simulink model "proc_control_lite"  (R2024b)
settings: Solver=FixedStepAuto  StartTime=0.0  StopTime=inf  RelTol=1e-3
InitFcn:
  | InitProcControl;
StartFcn:
  | LoadParams;
model workspace (MAT data in the model file):
  SL_ROS_VariableLengthArrays_MaxSizes.CommonInfo.ArrayTruncateAction = 'EmitWarning'
  SL_ROS_VariableLengthArrays_MaxSizes.MsgTypeMap = containers.Map
  SL_ROS_VariableLengthArrays_MaxSizes.MsgTypeMap.serialization.keys = {'sensor_msgs/Image', 'trajectory_msgs/MultiDOFJointTrajectoryPoint'}
  SL_ROS_VariableLengthArrays_MaxSizes.MsgTypeMap.serialization.values{1}(1).PropertyName = 'data'
  SL_ROS_VariableLengthArrays_MaxSizes.MsgTypeMap.serialization.values{1}(1).DataType = 'uint8'
  SL_ROS_VariableLengthArrays_MaxSizes.MsgTypeMap.serialization.values{1}(1).MaxLength = 2764800
  SL_ROS_VariableLengthArrays_MaxSizes.MsgTypeMap.serialization.values{1}(2).PropertyName = 'encoding'
  SL_ROS_VariableLengthArrays_MaxSizes.MsgTypeMap.serialization.values{1}(2).DataType = 'uint8'
  SL_ROS_VariableLengthArrays_MaxSizes.MsgTypeMap.serialization.values{1}(2).MaxLength = 128
  SL_ROS_VariableLengthArrays_MaxSizes.MsgTypeMap.serialization.values{2}(1).PropertyName = 'accelerations'
  SL_ROS_VariableLengthArrays_MaxSizes.MsgTypeMap.serialization.values{2}(1).DataType = 'geometry_msgs/Twist'
  SL_ROS_VariableLengthArrays_MaxSizes.MsgTypeMap.serialization.values{2}(1).MaxLength = 1024
  SL_ROS_VariableLengthArrays_MaxSizes.MsgTypeMap.serialization.values{2}(2).PropertyName = 'transforms'
  SL_ROS_VariableLengthArrays_MaxSizes.MsgTypeMap.serialization.values{2}(2).DataType = 'geometry_msgs/Transform'
  SL_ROS_VariableLengthArrays_MaxSizes.MsgTypeMap.serialization.values{2}(2).MaxLength = 1024
  SL_ROS_VariableLengthArrays_MaxSizes.MsgTypeMap.serialization.values{2}(3).PropertyName = 'velocities'
  SL_ROS_VariableLengthArrays_MaxSizes.MsgTypeMap.serialization.values{2}(3).DataType = 'geometry_msgs/Twist'
  SL_ROS_VariableLengthArrays_MaxSizes.MsgTypeMap.serialization.values{2}(3).MaxLength = 1024
  SL_ROS_VariableLengthArrays_MaxSizes.MsgTypeMap.serialization.uniformity = 0
  SL_ROS_VariableLengthArrays_MaxSizes.MsgTypeMap.serialization.keyType = 'char'
  SL_ROS_VariableLengthArrays_MaxSizes.MsgTypeMap.serialization.valueType = 'any'
values from neighbouring files (symbols this model uses):
  A = T200Spec16V{:,3}    [InitProcControl.m]
  N = T200Spec16V{:,6}    [InitProcControl.m]
  PWM = T200Spec16V{:,1}    [InitProcControl.m]
undefined symbols (not defined in the file or in its folder): config, current_gains, DiscIntNeverNeededParam, is_mpc_alive, is_trajectory_done, motor1, motor2, motor3, motor4, motor5, motor6, motor7, motor8, MPC, mpc_mode, mpc_status, orientation, physics, pose, position, simulation, simulink, target_reached, thrusters_status, thrusters_status_SL_Info, twist
libraries: ros2lib x64, dspstat3 x24, aerolibutil x15, dspfdesign x7, simulink x5, mpclib x3, matrix_library x3, robotcorelib x2, sharedtransform x1, sharedTrackingLibrary x1
(part 1 of 3)
settings Model: SimulationMode=accelerator  Creator=relat  LastModifiedBy=root
settings OptimizationCC: StrengthReduction=on  PassReuseOutputArgsAs=Individual arguments  ZeroExternalMemoryAtStartup=off  ZeroInternalMemoryAtStartup=off  EfficientFloat2IntCast=on  MaxStackSize=64  OptimizeBlockOrder=speed  MultiThreadedLoops=on  EfficientTunableParamExpr=on
settings DebuggingCC: ParameterTunabilityLossMsg=error
settings HardwareCC: ProdLargestAtomicInteger=Long  ProdLargestAtomicFloat=Double  ProdLongLongMode=on  ProdHWDeviceType=ARM Compatible->ARM 64-bit (LLP64)  TargetBitPerLong=64  TargetBitPerPointer=64  TargetBitPerSizeT=64  TargetBitPerPtrDiffT=64  TargetLargestAtomicFloat=Float  TargetIntDivRoundTo=Zero  TargetEndianess=LittleEndian  TargetWordSize=64  TargetHWDeviceType=AMD->x86-64 (Linux 64)  UseEmbeddedCoderFeatures=off
settings ModelReferenceCC: UpdateModelReferenceTargets=IfOutOfDate  EnableRefExpFcnMdlSchedulingChecks=on  EnableParallelModelReferenceBuilds=on
settings SFSimCC: SFSimEcho=off  MATLABDynamicMemAlloc=off  SimTargetLang=C++
settings RTWCC: Description=Embedded Coder  SystemTargetFile=ert.tlc  HardwareBoard=Robot Operating System 2 (ROS 2)  TLCOptions="-aInlineSetEventsForThisBaseRateFcn=TLC_FALSE -aSuppressMultiTaskScheduler=TLC_FALSE  -aRateBasedStepFcn=0"  GenCodeOnly=on  TemplateMakefile=ert_default_tmf  RetainRTWFile=on  Toolchain=Colcon Tools  BuildConfiguration=Faster Runs  TargetLang=C++
settings CodeAppCC: ForceParamTrailComments=on  IgnoreCustomStorageClasses=off  IgnoreTestpoints=on  OperatorAnnotations=on  SimulinkDataObjDesc=on  SFDataObjDesc=on  InsertBlockDesc=on
settings ERTTargetCC: TargetLangStandard=C++11 (ISO)  UtilityFuncGeneration=Shared location  CodeInterfacePackaging=C++ class  SupportNonInlinedSFcns=on  SupportVariableSizeSignals=on  InlinedParameterPlacement=Hierarchical  RootIOFormat=Structure reference  DynamicArrayContainerType=coder::array

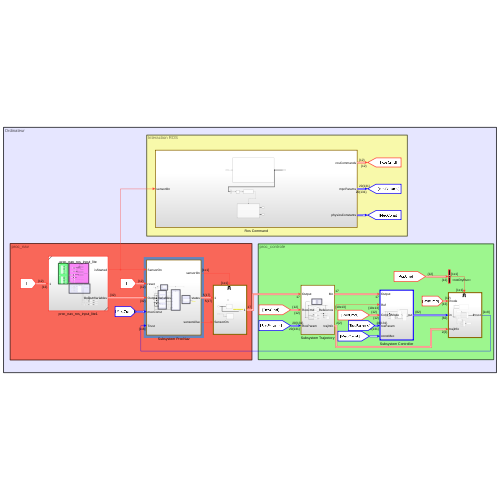
[thumbnail: Simulink's stored preview of the top-level diagram]
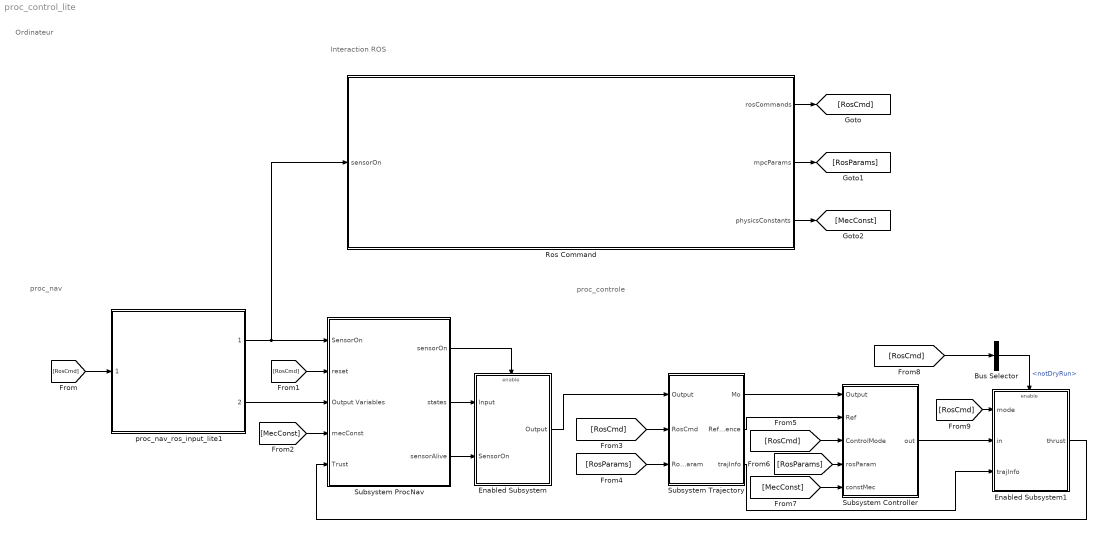
== system proc_control_lite ==
  note: Ordinateur
  note: proc_controle
  note: proc_nav
  note: Interaction ROS
  Bus Selector : BusSelector  OutputSignals=notDryRun
  Enabled Subsystem : Subsystem  TreatAsAtomicUnit=on
  Enabled Subsystem1 : Subsystem  TreatAsAtomicUnit=on
  Ros Command : Subsystem
  Subsystem Controller : Subsystem  TreatAsAtomicUnit=on  SystemSampleTime=MPC.Ts
  Subsystem ProcNav : Subsystem
  Subsystem Trajectory : Subsystem
  proc_nav_ros_input_lite1 : Subsystem  ReferencedSubsystem=proc_nav_ros_input_lite
  wires:
  Ros Command/1(rosCommands) -> [RosCmd]
  Ros Command/2(mpcParams) -> [RosParams]
  Ros Command/3(physicsConstants) -> [MecConst]
  [RosCmd] -> proc_nav_ros_input_lite1/1
  proc_nav_ros_input_lite1/1 -> Ros Command/1(sensorOn), Subsystem ProcNav/1(SensorOn)
  [RosCmd] -> Subsystem ProcNav/2(reset)
  proc_nav_ros_input_lite1/2 -> Subsystem ProcNav/3(Output Variables)
  [MecConst] -> Subsystem ProcNav/4(mecConst)
  Subsystem ProcNav/1(sensorOn) -> Enabled Subsystem/Enable
  Subsystem ProcNav/3(sensorAlive) -> Enabled Subsystem/2(SensorOn)
  [RosCmd] -> Subsystem Trajectory/2(RosCmd)
  [RosParams] -> Subsystem Trajectory/3(RosParam)
  Subsystem Trajectory/1(Mo) -> Subsystem Controller/1(Output)
  Subsystem Trajectory/2(Reference) -> Subsystem Controller/2(Ref)
  [RosCmd] -> Subsystem Controller/3(ControlMode)
  [RosParams] -> Subsystem Controller/4(rosParam)
  [MecConst] -> Subsystem Controller/5(constMec)
  Bus Selector/1 -> Enabled Subsystem1/Enable  "<notDryRun>"
  [RosCmd] -> Bus Selector/1
  [RosCmd] -> Enabled Subsystem1/1(mode)
  Subsystem Controller/1(out) -> Enabled Subsystem1/2(in)
  Subsystem Trajectory/3(trajInfo) -> Enabled Subsystem1/3(trajInfo)
  Enabled Subsystem1/1(thrust) -> Subsystem ProcNav/5(Trust)
  Subsystem ProcNav/2(states) -> Enabled Subsystem/1(Input)
  Enabled Subsystem/1(Output) -> Subsystem Trajectory/1(Output)

== system proc_control_lite/Enabled Subsystem ==
  note: Skipped Commented Blocks
  Input : Inport
  SensorOn : Inport  Port=2
  Enable : EnablePort
  Send Sensor On : Subsystem
  Send auv states : Subsystem
  Output : Outport
  wires:
  Input/1 -> Output/1, Send auv states/1(Input)
  SensorOn/1 -> Send Sensor On/1(IsReached)

== system proc_control_lite/Enabled Subsystem1 ==
  mode : Inport
  in : Inport  Port=2
  trajInfo : Inport  Port=3
  Enable : EnablePort
  Blank Message : ros2lib/Blank Message  messageClass=Message  entityType=sonia_common_ros2/MotorPwm  messageType=sonia_common_ros2/MotorPwm  SampleTime=inf
  Blank Message1 : ros2lib/Blank Message  messageClass=Message  entityType=sonia_common_ros2/MotorNewton  messageType=sonia_common_ros2/MotorNewton  SampleTime=inf
  Bus Assignment : BusAssignment  AssignedSignals=motor1,motor2,motor3,motor4,motor5,motor6,motor7,motor8
  Bus Assignment1 : BusAssignment  AssignedSignals=motor1,motor2,motor3,motor4,motor5,motor6,motor7,motor8
  Bus Selector : BusSelector  OutputSignals=mode
  Bus Selector1 : BusSelector  OutputSignals=pwm
  Bus Selector2 : BusSelector  OutputSignals=Newton
  Data Type Conversion : DataTypeConversion  OutDataTypeStr=single  SaturateOnIntegerOverflow=off  RndMeth=Floor
  Demux : Demux  Outputs=8
  Demux1 : Demux  Outputs=8
  Subsystem : Subsystem
  provider_thruster thruster_pwm : ros2lib/Publish  topicSource=Specify your own  topic=/provider_thruster/thruster_pwm  messageType=sonia_common_ros2/MotorPwm  QOSHistory=Keep last  QOSDepth=1  QOSReliability=Reliable  QOSDurability=Volatile  QOSDeadline=Inf  QOSLifespan=Inf  QOSLiveliness=Automatic  QOSLeaseDuration=Inf  QOSAvoidROSNamespaceConventions=off
  telemetry thruster_newton : ros2lib/Publish  topicSource=Specify your own  topic=/telemetry/thruster_newton  messageType=sonia_common_ros2/MotorNewton  QOSHistory=Keep last  QOSDepth=1  QOSReliability=Reliable  QOSDurability=Volatile  QOSDeadline=Inf  QOSLifespan=Inf  QOSLiveliness=Automatic  QOSLeaseDuration=Inf  QOSAvoidROSNamespaceConventions=off
  thrust : Outport
  wires:
  trajInfo/1 -> Subsystem/1(trajInfo)
  mode/1 -> Bus Selector/1
  in/1 -> Subsystem/3(mpc param), Bus Selector2/1, Bus Selector1/1
  Bus Selector1/1 -> Demux/1  "<pwm>"
  Bus Selector2/1 -> thrust/1, Data Type Conversion/1  "<Newton>"
  Blank Message/1 -> Bus Assignment/1
  Bus Assignment/1 -> provider_thruster thruster_pwm/1
  Bus Assignment1/1 -> telemetry thruster_newton/1
  Demux1/4 -> Bus Assignment1/5
  Demux1/1 -> Bus Assignment1/2
  Demux1/2 -> Bus Assignment1/3
  Blank Message1/1 -> Bus Assignment1/1
  Demux1/3 -> Bus Assignment1/4
  Demux1/5 -> Bus Assignment1/6
  Demux1/6 -> Bus Assignment1/7
  Demux1/7 -> Bus Assignment1/8
  Demux1/8 -> Bus Assignment1/9
  Data Type Conversion/1 -> Demux1/1
  Bus Selector/1 -> Subsystem/2(mode)  "<mode>"
  Demux/2 -> Bus Assignment/3
  Demux/3 -> Bus Assignment/4
  Demux/1 -> Bus Assignment/2
  Demux/4 -> Bus Assignment/5
  Demux/6 -> Bus Assignment/7
  Demux/5 -> Bus Assignment/6
  Demux/8 -> Bus Assignment/9
  Demux/7 -> Bus Assignment/8

== system proc_control_lite/Ros Command ==
  sensorOn : Inport
  Bus Selector : BusSelector  OutputSignals=mode
  Get_ROS_param : Subsystem  TreatAsAtomicUnit=on
  If : If  IfExpression=u1 == 0  ShowElse=off
  Ros Command Manager : Subsystem
  Zero-Order Hold : ZeroOrderHold  SampleTime=simulink.ros.paramSampletime
  rosCommands : Outport
  mpcParams : Outport  Port=2
  physicsConstants : Outport  Port=3
  wires:
  Ros Command Manager/1(rosCommands) -> rosCommands/1, Bus Selector/1
  Get_ROS_param/1(mpcParams) -> mpcParams/1
  Zero-Order Hold/1 -> If/1
  Bus Selector/1 -> Zero-Order Hold/1  "<mode>"
  If/1 -> Get_ROS_param/Action
  sensorOn/1 -> Ros Command Manager/1(sensorOn)
  Get_ROS_param/2(physicsConstants) -> physicsConstants/1

== system proc_control_lite/Subsystem Controller ==
  Output : Inport
  Ref : Inport  Port=2
  ControlMode : Inport  Port=3
  rosParam : Inport  Port=4
  constMec : Inport  Port=5
  Bus Selector : BusSelector  OutputSignals=mode
  Bus Selector1 : BusSelector  OutputSignals=current
  Controller List : Subsystem
  Delay : Delay  DelayLength=1  InitialCondition=zeros(1,8)  SampleTime=MPC.Ts
  If : If  IfExpression=u1 >= 0  ShowElse=off
  If Action Subsystem : Subsystem  TreatAsAtomicUnit=on
  Post Traitement : Subsystem
  out : Outport
  wires:
  Output/1 -> Controller List/1(mo), If Action Subsystem/2(mo)
  ControlMode/1 -> Bus Selector/1
  Bus Selector/1 -> Controller List/2(ControlMode), If Action Subsystem/1(mode), If/1  "<mode>"
  If/1 -> If Action Subsystem/Action
  rosParam/1 -> If Action Subsystem/4(mpcParams)
  If Action Subsystem/1(MPC param) -> Post Traitement/2(MpcParams), Controller List/4(mpc param)
  constMec/1 -> Controller List/5(constMec)
  Ref/1 -> Controller List/3(Ref)
  Controller List/1(Out1) -> Post Traitement/1(In1)
  Post Traitement/1(out) -> Bus Selector1/1, out/1
  Bus Selector1/1 -> Delay/1  "<current>"
  Delay/1 -> If Action Subsystem/3(Current)

== system proc_control_lite/Subsystem ProcNav ==
  note: Skipped Commented Block
  note: Mettre les données
      | dans un bus
  note: Filtre EKF
  note: Pre traitement des mesures
  note: Conditions pour activer le kalman
  SensorOn : Inport
  reset : Inport  Port=2
  Output Variables : Inport  Port=3
  mecConst : Inport  Port=4
  Trust : Inport  Port=5
  AHRS/Detph Mesurments : Subsystem
  Bus Selector : BusSelector  OutputSignals=navReset
  Bus Selector1 : BusSelector  OutputSignals=NewDvlMsg
  Bus Selector2 : BusSelector  OutputSignals=new Pressure Msg
  Constant : Constant  Commented=on  Value=false
  DVL Measurements : Subsystem  TreatAsAtomicUnit=on
  Delay : Delay  DelayLength=10  InitialConditionSource=Input port  InitialCondition=0
      settings: InputPortMap=u0,p4
  Depth Measurements : Subsystem  TreatAsAtomicUnit=on
  Enabled Subsystem : Subsystem  TreatAsAtomicUnit=on
  Reset Logic : Subsystem
  State function arguments : Subsystem
  mux2Bus : Subsystem
  sensorOn : Outport
  states : Outport  Port=2
  sensorAlive : Outport  Port=3
  wires:
  reset/1 -> Bus Selector/1
  Bus Selector/1 -> Reset Logic/1(In1)  "<navReset>"
  Reset Logic/1(Out1) -> Enabled Subsystem/Enable, sensorOn/1
  Trust/1 -> State function arguments/1(thrust)
  mecConst/1 -> State function arguments/2(mecConst), DVL Measurements/2(mecConst), Enabled Subsystem/6(mecConst), Depth Measurements/2(mecConst)
  Output Variables/1 -> DVL Measurements/1(DVL Velocity), Bus Selector2/1, Depth Measurements/1(y), Bus Selector1/1, AHRS/Detph Mesurments/1(y)
  Bus Selector1/1 -> DVL Measurements/Enable  "<NewDvlMsg>"
  Bus Selector2/1 -> Depth Measurements/Enable  "<new Pressure Msg>"
  AHRS/Detph Mesurments/1(IMU) -> Depth Measurements/3(xhat), Enabled Subsystem/2(AHRS Mesurments)
  State function arguments/1(stateFuncArguments) -> Enabled Subsystem/1(stateFuncArguments)
  DVL Measurements/1(DVL Measurements) -> Enabled Subsystem/4("DVL Measurements ")
  Depth Measurements/1(Depth Measurements) -> Enabled Subsystem/5(Depth Measurements)
  Enabled Subsystem/1(xhat) -> mux2Bus/1(xhat)
  mux2Bus/1(states) -> states/1  "md"
  AHRS/Detph Mesurments/2(ZED) -> Enabled Subsystem/3(ZED)
  SensorOn/1 -> Delay/2, AHRS/Detph Mesurments/2(SensorOn), Delay/1
  Delay/1 -> Reset Logic/2(2), sensorAlive/1

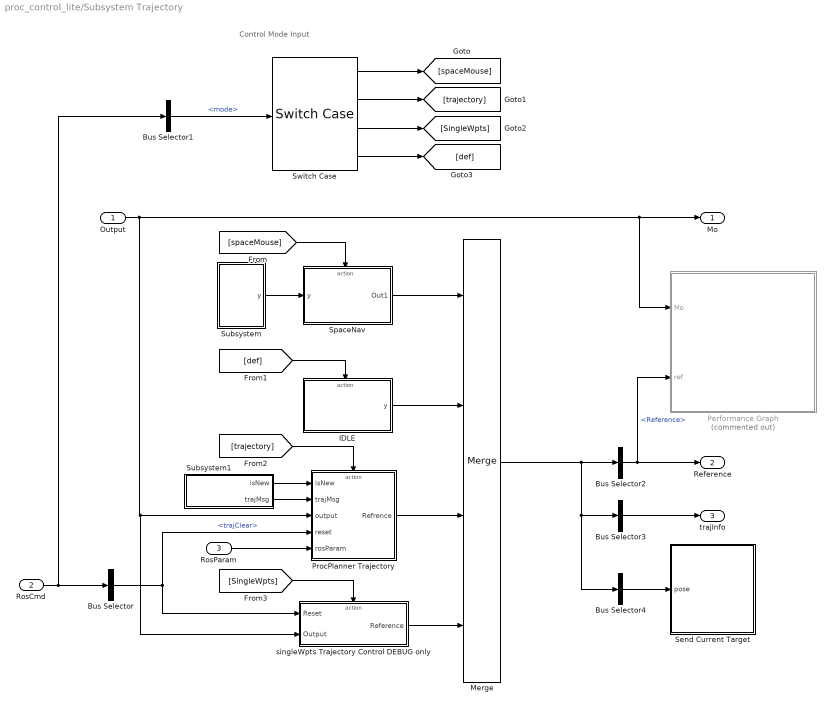
== system proc_control_lite/Subsystem Trajectory ==
  note: Control Mode Input
  Output : Inport
  RosCmd : Inport  Port=2
  RosParam : Inport  Port=3
  Bus Selector : BusSelector  OutputSignals=trajClear
  Bus Selector1 : BusSelector  OutputSignals=mode
  Bus Selector2 : BusSelector  OutputSignals=Reference
  Bus Selector3 : BusSelector  OutputSignals=isReached,isTrajDone  OutputAsBus=on
  Bus Selector4 : BusSelector  OutputSignals=target  OutputAsBus=on
  IDLE : Subsystem  TreatAsAtomicUnit=on
  Merge : Merge  Inputs=4
  Performance Graph : Subsystem  Commented=on
  ProcPlanner Trajectory : Subsystem  TreatAsAtomicUnit=on
  Send Current Target : Subsystem
  SpaceNav : Subsystem  TreatAsAtomicUnit=on
  Subsystem : Subsystem
  Subsystem1 : Subsystem
  Switch Case : SwitchCase  CaseConditions={mode.traj.SpaceMouseMode,mode.traj.trajMode, mode.traj.singleWpts,}
  singleWpts Trajectory Control DEBUG only : Subsystem  TreatAsAtomicUnit=on
  Mo : Outport
  Reference : Outport  Port=2
  trajInfo : Outport  Port=3
  wires:
  RosCmd/1 -> Bus Selector1/1, Bus Selector/1
  Bus Selector1/1 -> Switch Case/1  "<mode>"
  Switch Case/1 -> [spaceMouse]
  Switch Case/2 -> [trajectory]
  Switch Case/3 -> [SingleWpts]
  Switch Case/4 -> [def]
  Output/1 -> singleWpts Trajectory Control DEBUG only/2(Output), ProcPlanner Trajectory/3(output), Performance Graph/1(Mo), Mo/1
  [spaceMouse] -> SpaceNav/Action
  Subsystem/1(y) -> SpaceNav/1(y)
  [def] -> IDLE/Action
  [trajectory] -> ProcPlanner Trajectory/Action
  Subsystem1/1(isNew) -> ProcPlanner Trajectory/1(isNew)
  Subsystem1/2(trajMsg) -> ProcPlanner Trajectory/2(trajMsg)
  Bus Selector/1 -> singleWpts Trajectory Control DEBUG only/1(Reset), ProcPlanner Trajectory/4(reset)  "<trajClear>"
  RosParam/1 -> ProcPlanner Trajectory/5(rosParam)
  [SingleWpts] -> singleWpts Trajectory Control DEBUG only/Action
  SpaceNav/1(Out1) -> Merge/1
  IDLE/1(y) -> Merge/2
  ProcPlanner Trajectory/1(Refrence) -> Merge/3
  singleWpts Trajectory Control DEBUG only/1(Reference) -> Merge/4
  Merge/1 -> Bus Selector4/1, Bus Selector3/1, Bus Selector2/1
  Bus Selector2/1 -> Performance Graph/2(ref), Reference/1  "<Reference>"
  Bus Selector3/1 -> trajInfo/1
  Bus Selector4/1 -> Send Current Target/1(pose)

== system proc_control_lite/Enabled Subsystem/Send Sensor On ==
  IsReached : Inport
  Blank Message : ros2lib/Blank Message  messageClass=Message  entityType=std_msgs/Bool  messageType=std_msgs/Bool  SampleTime=inf
  Bus Assignment : BusAssignment  AssignedSignals=data
  Data Type Conversion : DataTypeConversion  OutDataTypeStr=boolean  SaturateOnIntegerOverflow=off  RndMeth=Floor
  Zero-Order Hold : ZeroOrderHold
  proc_control sensor_on : ros2lib/Publish  topicSource=Specify your own  topic=/proc_control/sensor_on  messageType=std_msgs/Bool  QOSHistory=Keep last  QOSDepth=1  QOSReliability=Reliable  QOSDurability=Volatile  QOSDeadline=Inf  QOSLifespan=Inf  QOSLiveliness=Automatic  QOSLeaseDuration=Inf  QOSAvoidROSNamespaceConventions=off
  wires:
  Bus Assignment/1 -> Zero-Order Hold/1
  Zero-Order Hold/1 -> proc_control sensor_on/1
  Data Type Conversion/1 -> Bus Assignment/2
  Blank Message/1 -> Bus Assignment/1
  IsReached/1 -> Data Type Conversion/1

== system proc_control_lite/Enabled Subsystem/Send auv states ==
  Input : Inport
  Blank Message : ros2lib/Blank Message  messageClass=Message  entityType=nav_msgs/Odometry  messageType=nav_msgs/Odometry  SampleTime=inf
  Bus Assignment : BusAssignment  AssignedSignals=pose.pose.position.x,pose.pose.position.y,pose.pose.position.z,pose.pose.orientation.w,pose.pose.orientation.x,pose.pose.orientation.y,pose.pose.orientation.z,twist.twist.linear.x,twist.twist.linear.y,twist.twist.linear.z,twist.twist.angular.x,twist.twist.angular.y,twist.twist.angular.z
  Demux : Demux  Outputs=13
  Header Assignment : ros2lib/Header Assignment  SetFrameID=on  FrameID=NED  InsertTimeStamp=on  SetHeaderFieldName=Use the default header field name  HeaderFieldName=header
  bus2mux : Subsystem
  proc_nav auv_states : ros2lib/Publish  topicSource=Specify your own  topic=/proc_nav/auv_states  messageType=nav_msgs/Odometry  QOSHistory=Keep last  QOSDepth=1  QOSReliability=Reliable  QOSDurability=Volatile  QOSDeadline=Inf  QOSLifespan=5  QOSLiveliness=Automatic  QOSLeaseDuration=5  QOSAvoidROSNamespaceConventions=off
  wires:
  Blank Message/1 -> Header Assignment/1
  Input/1 -> bus2mux/1(Input)
  Header Assignment/1 -> Bus Assignment/1
  bus2mux/1(states) -> Demux/1
  Demux/1 -> Bus Assignment/2
  Demux/2 -> Bus Assignment/3
  Demux/3 -> Bus Assignment/4
  Demux/4 -> Bus Assignment/5
  Demux/5 -> Bus Assignment/6
  Demux/6 -> Bus Assignment/7
  Demux/7 -> Bus Assignment/8
  Demux/8 -> Bus Assignment/9
  Demux/9 -> Bus Assignment/10
  Demux/10 -> Bus Assignment/11
  Demux/11 -> Bus Assignment/12
  Demux/12 -> Bus Assignment/13
  Demux/13 -> Bus Assignment/14
  Bus Assignment/1 -> proc_nav auv_states/1

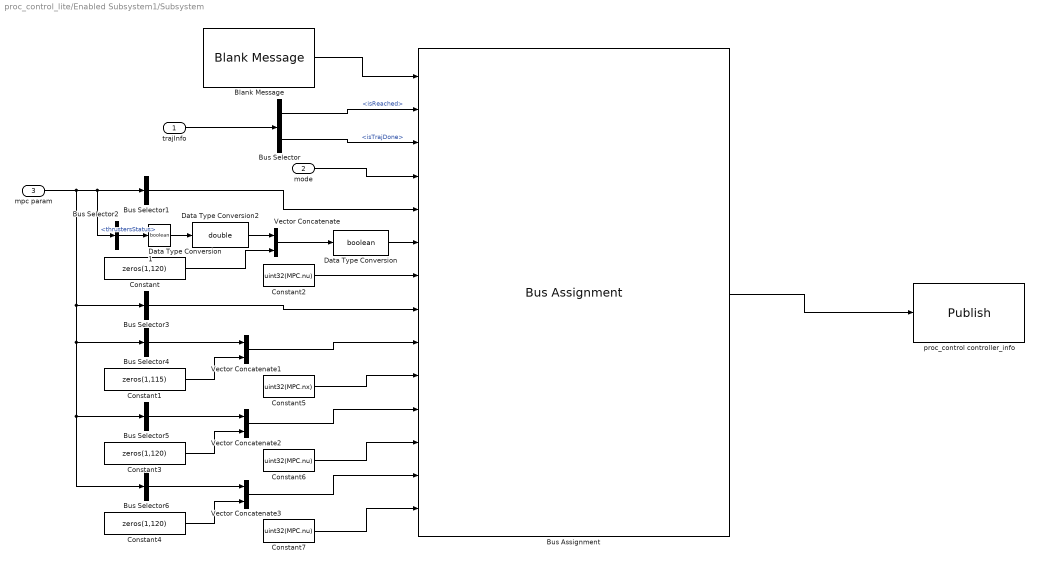
== system proc_control_lite/Enabled Subsystem1/Subsystem ==
  trajInfo : Inport
  mode : Inport  Port=2
  mpc param : Inport  Port=3  SampleTime=0.02
  Blank Message : ros2lib/Blank Message  messageClass=Message  entityType=sonia_common_ros2/MpcInfo  messageType=sonia_common_ros2/MpcInfo  SampleTime=inf
  Bus Assignment : BusAssignment  AssignedSignals=target_reached,is_trajectory_done,mpc_mode,is_mpc_alive,thrusters_status,thrusters_status_SL_Info.CurrentLength,mpc_status,current_gains.ov,current_gains.ov_SL_Info.CurrentLength,current_gains.mv,current_gains.mv_SL_Info.CurrentLength,current_gains.mvr,current_gains.mvr_SL_Info.CurrentLength
  Bus Selector : BusSelector  OutputSignals=isReached,isTrajDone
  Bus Selector1 : BusSelector  OutputSignals=isMpcAlive  OutputAsBus=on
  Bus Selector2 : BusSelector  OutputSignals=mpcParams.thrustersStatus
  Bus Selector3 : BusSelector  OutputSignals=MpcStatus  OutputAsBus=on
  Bus Selector4 : BusSelector  OutputSignals=mpcParams.ywt  OutputAsBus=on
  Bus Selector5 : BusSelector  OutputSignals=mpcParams.mvwt  OutputAsBus=on
  Bus Selector6 : BusSelector  OutputSignals=mpcParams.dmwwt  OutputAsBus=on
  Constant : Constant  Value=zeros(1,120)  VectorParams1D=off
  Constant1 : Constant  Value=zeros(1,115)  VectorParams1D=off
  Constant2 : Constant  Value=uint32(MPC.nu)
  Constant3 : Constant  Value=zeros(1,120)  VectorParams1D=off
  Constant4 : Constant  Value=zeros(1,120)  VectorParams1D=off
  Constant5 : Constant  Value=uint32(MPC.nx)  VectorParams1D=off
  Constant6 : Constant  Value=uint32(MPC.nu)
  Constant7 : Constant  Value=uint32(MPC.nu)
  Data Type Conversion : DataTypeConversion  OutDataTypeStr=boolean  SaturateOnIntegerOverflow=off  RndMeth=Floor
  Data Type Conversion1 : DataTypeConversion  OutDataTypeStr=boolean  SaturateOnIntegerOverflow=off  RndMeth=Floor
  Data Type Conversion2 : DataTypeConversion  OutDataTypeStr=double  SaturateOnIntegerOverflow=off  RndMeth=Floor
  Vector Concatenate{,1..3} (4 alike) : Concatenate
  proc_control controller_info : ros2lib/Publish  topicSource=Specify your own  topic=proc_control/controller_info  messageType=sonia_common_ros2/MpcInfo  QOSHistory=Keep last  QOSDepth=1  QOSReliability=Reliable  QOSDurability=Volatile  QOSDeadline=Inf  QOSLifespan=Inf  QOSLiveliness=Automatic  QOSLeaseDuration=Inf  QOSAvoidROSNamespaceConventions=off
  wires:
  Constant7/1 -> Bus Assignment/14
  Vector Concatenate3/1 -> Bus Assignment/13
  Constant6/1 -> Bus Assignment/12
  Vector Concatenate2/1 -> Bus Assignment/11
  Constant5/1 -> Bus Assignment/10
  Vector Concatenate1/1 -> Bus Assignment/9
  Constant2/1 -> Bus Assignment/7
  Vector Concatenate/1 -> Data Type Conversion/1
  Bus Selector/2 -> Bus Assignment/3  "<isTrajDone>"
  mpc param/1 -> Bus Selector6/1, Bus Selector5/1, Bus Selector4/1, Bus Selector3/1, Bus Selector2/1, Bus Selector1/1
  mode/1 -> Bus Assignment/4
  trajInfo/1 -> Bus Selector/1
  Constant3/1 -> Vector Concatenate2/2
  Bus Selector4/1 -> Vector Concatenate1/1
  Bus Selector2/1 -> Data Type Conversion1/1  "<thrustersStatus>"
  Bus Selector6/1 -> Vector Concatenate3/1
  Constant/1 -> Vector Concatenate/2
  Bus Selector3/1 -> Bus Assignment/8
  Bus Selector1/1 -> Bus Assignment/5
  Constant1/1 -> Vector Concatenate1/2
  Bus Selector/1 -> Bus Assignment/2  "<isReached>"
  Bus Selector5/1 -> Vector Concatenate2/1
  Constant4/1 -> Vector Concatenate3/2
  Blank Message/1 -> Bus Assignment/1
  Data Type Conversion/1 -> Bus Assignment/6
  Data Type Conversion1/1 -> Data Type Conversion2/1
  Data Type Conversion2/1 -> Vector Concatenate/1
  Bus Assignment/1 -> proc_control controller_info/1

== system proc_control_lite/Ros Command/Get_ROS_param ==
  Action Port : ActionPort  InitializeStates=reset  ActionPortLabel=if(u1 == 0)
  MPC Parameters : Subsystem
  Physics Constants : Subsystem
  mpcParams : Outport
  physicsConstants : Outport  Port=2
  wires:
  Physics Constants/1(physicsConstants) -> physicsConstants/1
  MPC Parameters/1(mpcParams) -> mpcParams/1

== system proc_control_lite/Ros Command/Ros Command Manager ==
  note: CUSTOM MESSAGE
  sensorOn : Inport
  Bus Creator : BusCreator  Inputs=7
  Bus Selector : BusSelector  OutputSignals=data  OutputAsBus=on
  Bus Selector1 : BusSelector  OutputSignals=data  OutputAsBus=on
  Bus Selector2 : BusSelector  OutputSignals=status  OutputAsBus=on
  Bus Selector3 : BusSelector  OutputSignals=position,orientation  OutputAsBus=on
  Bus Selector4 : BusSelector  OutputSignals=data  OutputAsBus=on
  Data Type Conversion : DataTypeConversion  OutDataTypeStr=uint8  SaturateOnIntegerOverflow=off  RndMeth=Floor
  Delay : Delay  DelayLength=1  InitialCondition=0
  MATLAB System : MATLABSystem  System=rosCommandManager  initial_mode=mode.init  SimulateUsing=Code generation
      mask Type: rosCommandManager
      mask Display:
      | disp('rosCommandManager');
      | port_label('input',1,'newSetMode');
      | port_label('input',2,'setMode');
      | port_label('input',3,'newReset');
      | port_label('input',4,'reset');
      | port_label('input',5,'newKill');
      | port_label('input',6,'kill');
      | port_label('input',7,'newIc');
      | port_label('input',8,'ic');
      | port_label('input',9,'newDryRun');
      | port_label('input',10,'Dryrun');
      | port_label('input',11,'newTrajreset');
      | port_label('input',12,'sensorOn');
      | port_label('output',1,'initQuat');
      | port_label('output',2,'initPos');
      | port_label('output',3,'simEnable');
      | port_label('output',4,'reset');
      | port_label('output',5,'mode');
      | port_label('output',6,'trajClear');
      | port_label('output',7,'notDryRun');
  Terminator : Terminator
  proc_control reset_trajectory : ros2lib/Subscribe  topicSource=Specify your own  topic=/proc_control/reset_trajectory  messageType=std_msgs/Bool  sampleTime=MPC.Ts  QOSHistory=Keep last  QOSDepth=10  QOSReliability=Reliable  QOSDurability=Volatile  QOSDeadline=inf  QOSLifespan=inf  QOSLiveliness=Automatic  QOSLeaseDuration=inf  QOSAvoidROSNamespaceConventions=off
  proc_control set_mode : ros2lib/Subscribe  topicSource=Specify your own  topic=/proc_control/set_mode  messageType=std_msgs/UInt8  sampleTime=MPC.Ts  QOSHistory=Keep last  QOSDepth=10  QOSReliability=Reliable  QOSDurability=Volatile  QOSDeadline=inf  QOSLifespan=inf  QOSLiveliness=Automatic  QOSLeaseDuration=inf  QOSAvoidROSNamespaceConventions=off
  proc_nav reset_pos : ros2lib/Subscribe  topicSource=Specify your own  topic=/proc_nav/reset_pos  messageType=std_msgs/Bool  sampleTime=MPC.Ts  QOSHistory=Keep last  QOSDepth=1  QOSReliability=Reliable  QOSDurability=Volatile  QOSDeadline=Inf  QOSLifespan=Inf  QOSLiveliness=Automatic  QOSLeaseDuration=Inf  QOSAvoidROSNamespaceConventions=off
  proc_simulation start_simulation : ros2lib/Subscribe  topicSource=Specify your own  topic=/proc_simulation/start_simulation  messageType=geometry_msgs/Pose  sampleTime=MPC.Ts  QOSHistory=Keep last  QOSDepth=10  QOSReliability=Reliable  QOSDurability=Volatile  QOSDeadline=inf  QOSLifespan=inf  QOSLiveliness=Automatic  QOSLeaseDuration=inf  QOSAvoidROSNamespaceConventions=off
  provider_rs485 kill_status : ros2lib/Subscribe  topicSource=Specify your own  topic=/provider_rs485/kill_status  messageType=sonia_common_ros2/KillStatus  sampleTime=MPC.Ts  QOSHistory=Keep last  QOSDepth=10  QOSReliability=Reliable  QOSDurability=Volatile  QOSDeadline=inf  QOSLifespan=inf  QOSLiveliness=Automatic  QOSLeaseDuration=inf  QOSAvoidROSNamespaceConventions=off
  telemetry dryrun : ros2lib/Subscribe  topicSource=Specify your own  topic=/telemetry/dry_run  messageType=std_msgs/Bool  sampleTime=MPC.Ts  QOSHistory=Keep last  QOSDepth=10  QOSReliability=Reliable  QOSDurability=Volatile  QOSDeadline=inf  QOSLifespan=inf  QOSLiveliness=Automatic  QOSLeaseDuration=inf  QOSAvoidROSNamespaceConventions=off
  rosCommands : Outport
  wires:
  Bus Selector1/1 -> MATLAB System/4
  Bus Selector4/1 -> MATLAB System/10
  MATLAB System/6 -> Bus Creator/6  "trajClear"
  Bus Selector2/1 -> MATLAB System/6
  MATLAB System/1 -> Bus Creator/1  "initQuat"
  MATLAB System/7 -> Bus Creator/7  "notDryRun"
  MATLAB System/4 -> Bus Creator/4  "navReset"
  Data Type Conversion/1 -> Bus Creator/5  "mode"
  MATLAB System/5 -> Data Type Conversion/1
  MATLAB System/3 -> Bus Creator/3  "simActivate"
  Bus Creator/1 -> rosCommands/1
  Delay/1 -> MATLAB System/12
  sensorOn/1 -> Delay/1
  MATLAB System/2 -> Bus Creator/2  "initPos"
  Bus Selector/1 -> MATLAB System/2
  Bus Selector3/1 -> MATLAB System/8
  proc_control set_mode/1 -> MATLAB System/1
  proc_control set_mode/2 -> Bus Selector/1
  proc_nav reset_pos/1 -> MATLAB System/3
  proc_nav reset_pos/2 -> Bus Selector1/1
  provider_rs485 kill_status/1 -> MATLAB System/5
  provider_rs485 kill_status/2 -> Bus Selector2/1
  proc_simulation start_simulation/1 -> MATLAB System/7
  proc_simulation start_simulation/2 -> Bus Selector3/1
  telemetry dryrun/1 -> MATLAB System/9
  telemetry dryrun/2 -> Bus Selector4/1
  proc_control reset_trajectory/1 -> MATLAB System/11
  proc_control reset_trajectory/2 -> Terminator/1

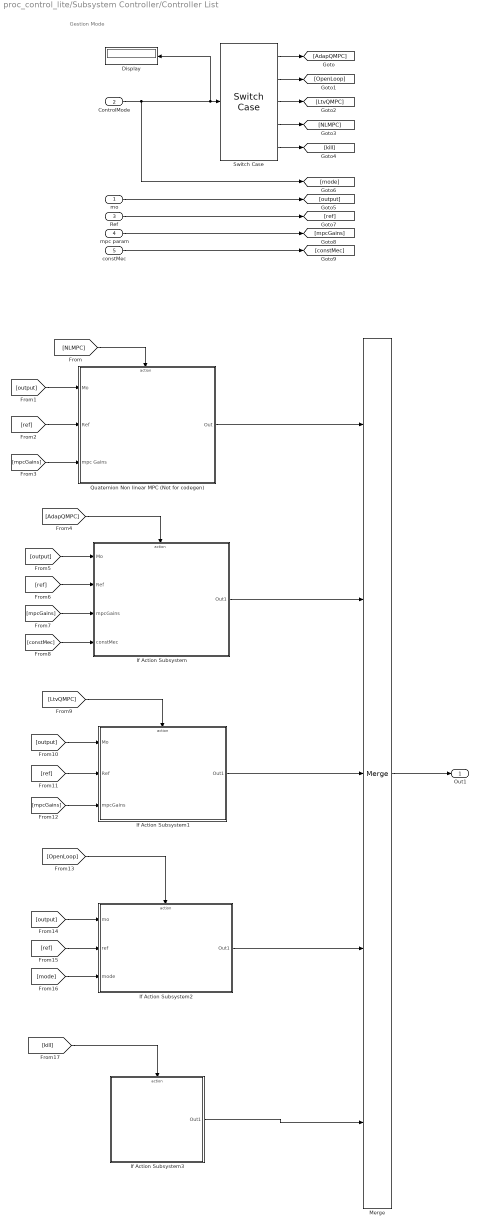
== system proc_control_lite/Subsystem Controller/Controller List ==
  note: Gestion Mode
  mo : Inport
  ControlMode : Inport  Port=2  SampleTime=MPC.Ts
  Ref : Inport  Port=3
  mpc param : Inport  Port=4
  constMec : Inport  Port=5
  Display : Display
  If Action Subsystem : Subsystem  TreatAsAtomicUnit=on
  If Action Subsystem1 : Subsystem  TreatAsAtomicUnit=on
  If Action Subsystem2 : Subsystem  TreatAsAtomicUnit=on
  If Action Subsystem3 : Subsystem  TreatAsAtomicUnit=on
  Merge : Merge  Inputs=5
  Quaternion Non linear MPC (Not for codegen) : Subsystem  TreatAsAtomicUnit=on
  Switch Case : SwitchCase  CaseConditions="{ mode.control.adapQMpcMode,  mode.control.openLoopMode,    mode.control.LtvQMpcMode, mode.control.NlmpcMode}"
  Out1 : Outport
  wires:
  ControlMode/1 -> [mode], Display/1, Switch Case/1
  Switch Case/1 -> [AdapQMPC]
  Switch Case/2 -> [OpenLoop]
  Switch Case/3 -> [LtvQMPC]
  Switch Case/4 -> [NLMPC]
  Switch Case/5 -> [kill]
  mo/1 -> [output]
  Ref/1 -> [ref]
  mpc param/1 -> [mpcGains]
  constMec/1 -> [constMec]
  [NLMPC] -> Quaternion Non linear MPC (Not for codegen)/Action
  [output] -> Quaternion Non linear MPC (Not for codegen)/1(Mo)
  [ref] -> Quaternion Non linear MPC (Not for codegen)/2(Ref)
  [mpcGains] -> Quaternion Non linear MPC (Not for codegen)/3(mpc Gains)
  [AdapQMPC] -> If Action Subsystem/Action
  [output] -> If Action Subsystem/1(Mo)
  [mpcGains] -> If Action Subsystem/3(mpcGains)
  [ref] -> If Action Subsystem/2(Ref)
  [constMec] -> If Action Subsystem/4(constMec)
  If Action Subsystem/1(Out1) -> Merge/2
  Quaternion Non linear MPC (Not for codegen)/1(Out) -> Merge/1
  Merge/1 -> Out1/1
  [LtvQMPC] -> If Action Subsystem1/Action
  [output] -> If Action Subsystem1/1(Mo)
  [ref] -> If Action Subsystem1/2(Ref)
  [mpcGains] -> If Action Subsystem1/3(mpcGains)
  If Action Subsystem1/1(Out1) -> Merge/3
  [OpenLoop] -> If Action Subsystem2/Action
  [mode] -> If Action Subsystem2/3(mode)
  [output] -> If Action Subsystem2/1(mo)
  [ref] -> If Action Subsystem2/2(ref)
  If Action Subsystem2/1(Out1) -> Merge/4
  [kill] -> If Action Subsystem3/Action
  If Action Subsystem3/1(Out1) -> Merge/5

== system proc_control_lite/Subsystem Controller/If Action Subsystem ==
  mode : Inport
  mo : Inport  Port=2
  Current : Inport  Port=3
  mpcParams : Inport  Port=4
  Action Port : ActionPort  InitializeStates=reset  ActionPortLabel=if(u1 >= 0)
  Bus Creator : BusCreator  Inputs=9
  Bus Selector : BusSelector  OutputSignals=qS2W
  Bus Selector1 : BusSelector  OutputSignals=data
  Constant : Constant  Commented=on  Value=false
  MATLAB System : MATLABSystem  System=mpcManager  mpcConst=MPC  mode=mode  SimulateUsing=Code generation
      mask Type: mpcManager
      mask Display:
      | disp('mpcManager');
      | port_label('input',1,'newRosGains');
      | port_label('input',2,'rosGains');
      | port_label('input',3,'mode');
      | port_label('input',4,'newReadCurrent');
      | port_label('input',5,'readCurrent');
      | port_label('input',6,'estimatedCurrent');
      | port_label('input',7,'mo');
      | port_label('input',8,'mpcParams');
      | port_label('output',1,'mvmin');
      | port_label('output',2,'mvmax');
      | port_label('output',3,'ywt');
      | port_label('output',4,'mvwt');
      | port_label('output',5,'dmwwt');
      | port_label('output',6,'tInfo');
      | port_label('output',7,'kill');
      | port_label('output',8,'p');
      | port_label('output',9,'m');
  Subscribe : ros2lib/Subscribe  topicSource=Specify your own  topic=/proc_control/set_mpc_gains  messageType=sonia_common_ros2/MpcGains  sampleTime=inf  QOSHistory=Keep last  QOSDepth=1  QOSReliability=Reliable  QOSDurability=Volatile  QOSDeadline=5  QOSLifespan=5  QOSLiveliness=Automatic  QOSLeaseDuration=5  QOSAvoidROSNamespaceConventions=off
  Subscribe1 : ros2lib/Subscribe  topicSource=Specify your own  topic=/provider_power/current_not  messageType=std_msgs/Float64MultiArray  sampleTime=-1  QOSHistory=Keep last  QOSDepth=1  QOSReliability=Reliable  QOSDurability=Volatile  QOSDeadline=5  QOSLifespan=5  QOSLiveliness=Automatic  QOSLeaseDuration=5  QOSAvoidROSNamespaceConventions=off
  Subsystem : Subsystem  Commented=on
  Transpose : Math  Operator=transpose
  MPC param : Outport
  wires:
  mode/1 -> MATLAB System/3
  Current/1 -> MATLAB System/6
  mo/1 -> Bus Selector/1
  Transpose/1 -> MATLAB System/5
  Bus Selector1/1 -> Transpose/1  "<data>"
  Bus Selector/1 -> MATLAB System/7  "<qS2W>"
  MATLAB System/1 -> Bus Creator/1  "mvmin"
  MATLAB System/2 -> Bus Creator/2  "mvmax"
  MATLAB System/3 -> Bus Creator/3  "ywt"
  MATLAB System/4 -> Bus Creator/4  "mvwt"
  MATLAB System/5 -> Bus Creator/5  "dmwwt"
  MATLAB System/6 -> Bus Creator/6  "thrustersStatus"
  MATLAB System/7 -> Bus Creator/7  "kill"
  MATLAB System/8 -> Bus Creator/8  "p"
  MATLAB System/9 -> Bus Creator/9  "m"
  Bus Creator/1 -> MPC param/1
  mpcParams/1 -> MATLAB System/8
  Subscribe1/2 -> Bus Selector1/1  "data"
  Subscribe1/1 -> MATLAB System/4
  Subscribe/2 -> MATLAB System/2
  Subscribe/1 -> MATLAB System/1

== system proc_control_lite/Subsystem Controller/Post Traitement ==
  In1 : Inport
  MpcParams : Inport  Port=2
  Bus Creator : BusCreator  Inputs=6
  Bus Selector : BusSelector  OutputSignals=mv
  Bus Selector1 : BusSelector  OutputSignals=mvmax,mvmin
  Bus Selector2 : BusSelector  OutputSignals=MpcStatus
  Bus Selector3 : BusSelector  OutputSignals=alive
  Data Type Conversion : DataTypeConversion  OutDataTypeStr=boolean  SaturateOnIntegerOverflow=off  RndMeth=Floor
  Delay : Delay  DelayLength=1  SampleTime=MPC.Ts
  N to A : Lookup_n-D  NumberOfTableDimensions=1  BreakpointsForDimension1=N  BreakpointsForDimension3=[5, 7]  BeginIndexSearchUsingPreviousIndexResult=on  Table=A  InterpMethod=Nearest  DiagnosticForOutOfRangeInput=Warning  RemoveProtectionInput=on  InternalRulePriority=Speed  OutDataTypeStr=uint16  RndMeth=Simplest
  PSU Safe : simulink/Discontinuities/Saturation Dynamic  OutMin=[]  OutMax=[]  OutDataTypeStr=Inherit: Same as second input  OutDataType=fixdt(1, 16)  OutScaling=2^-10  DoSatur=off
  Sum : Sum  Inputs=|+-
  Transpose : Math  Operator=transpose
  n-D Lookup Table1 : Lookup_n-D  NumberOfTableDimensions=1  BreakpointsForDimension1=N  BreakpointsForDimension3=[5, 7]  BeginIndexSearchUsingPreviousIndexResult=on  Table=PWM  InterpMethod=Nearest  DiagnosticForOutOfRangeInput=Warning  RemoveProtectionInput=on  InternalRulePriority=Speed  OutDataTypeStr=uint16  RndMeth=Simplest
  out : Outport
  wires:
  In1/1 -> Bus Selector3/1, Bus Selector2/1, Bus Selector/1
  Bus Selector/1 -> Transpose/1  "<mv>"
  Transpose/1 -> PSU Safe/2
  Bus Selector1/1 -> PSU Safe/1  "<mvmax>"
  Bus Selector1/2 -> PSU Safe/3  "<mvmin>"
  PSU Safe/1 -> N to A/1, n-D Lookup Table1/1, Bus Creator/3  "Newton"
  n-D Lookup Table1/1 -> Bus Creator/2  "pwm"
  N to A/1 -> Bus Creator/1  "current"
  MpcParams/1 -> Bus Creator/4, Bus Selector1/1  "mpcParams"
  Bus Selector2/1 -> Bus Creator/5  "<MpcStatus>"
  Bus Selector3/1 -> Sum/2, Delay/1  "<alive>"
  Delay/1 -> Sum/1
  Sum/1 -> Data Type Conversion/1
  Data Type Conversion/1 -> Bus Creator/6  "isMpcAlive"
  Bus Creator/1 -> out/1

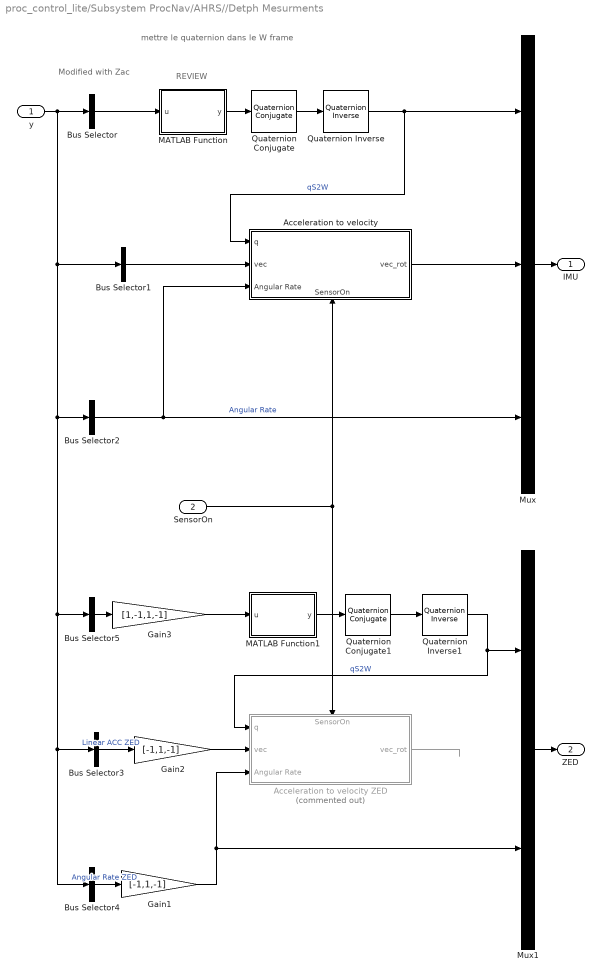
== system proc_control_lite/Subsystem ProcNav/AHRS//Detph Mesurments ==
  note: Modified with Zac
  note: REVIEW
  note: mettre le quaternion dans
      | le W frame
  y : Inport
  SensorOn : Inport  Port=2
  Acceleration to velocity : Subsystem  Variant=on  AllowZeroVariantControls=on
      settings: PortSchema="{\"entries\":[{\"content\":{\"sides\":[{\"content\":{\"connectorIds\":[\"In1\",\"In2\",\"In3\"]},\"type\":\"ConnectorPlacement.EquallySpacedRectSide\",\"uuid\":\"af4febd0-38b2-41fa-a6f4-f4ba4fe07e99\"},{\"content\":{\"connectorIds\":[\"Out1\"],\"side\":\"RIGHT\"},\"type\":\"ConnectorPlacement.EquallySpacedRectSide\",\"uuid\":\"0eb4adac-0140-4294-9ebb-74b685dc8d2b\"},{\"content\":{\"side\":\"TOP\"},\"type\":\"ConnectorPlacement.EquallySpacedRectSide\",\"uuid\":\"f5ce0cde-beaa-4ea1-adb5-998f154101aa\"},{\"content\":{\"connectorIds\":[\"In4\"],\"side\":\"BOTTOM\"},\"type\":\"ConnectorPlacement.EquallySpacedRectSide\",\"uuid\":\"93cbe6c9-6811-4450-85d4-79008a364440\"}]},\"type\":\"ConnectorPlacement.EquallySpacedConnector\",\"uuid\":\"367d0f59-ae10-4235-a592-a2cfb09d42c6\"}],\"packageUris\":[\"http://schema.mathworks.com/mf0/Connector/R2020b\"],\"version\":\"1.0\"}"
  Acceleration to velocity ZED : Subsystem  Commented=on  Variant=on  AllowZeroVariantControls=on
      settings: PortSchema="{\"entries\":[{\"content\":{\"sides\":[{\"content\":{\"connectorIds\":[\"In1\",\"In2\",\"In3\"]},\"type\":\"ConnectorPlacement.EquallySpacedRectSide\",\"uuid\":\"af4febd0-38b2-41fa-a6f4-f4ba4fe07e99\"},{\"content\":{\"connectorIds\":[\"Out1\"],\"side\":\"RIGHT\"},\"type\":\"ConnectorPlacement.EquallySpacedRectSide\",\"uuid\":\"0eb4adac-0140-4294-9ebb-74b685dc8d2b\"},{\"content\":{\"connectorIds\":[\"In4\"],\"side\":\"TOP\"},\"type\":\"ConnectorPlacement.EquallySpacedRectSide\",\"uuid\":\"f5ce0cde-beaa-4ea1-adb5-998f154101aa\"}]},\"type\":\"ConnectorPlacement.EquallySpacedConnector\",\"uuid\":\"367d0f59-ae10-4235-a592-a2cfb09d42c6\"}],\"packageUris\":[\"http://schema.mathworks.com/mf0/Connector/R2020b\"],\"version\":\"1.0\"}"
  Bus Selector : BusSelector  OutputSignals=Quaternion  OutputAsBus=on
  Bus Selector1 : BusSelector  OutputSignals=Linear Acc  OutputAsBus=on
  Bus Selector2 : BusSelector  OutputSignals=Angular Rate  OutputAsBus=on
  Bus Selector3 : BusSelector  OutputSignals=Linear Acc ZED  OutputAsBus=on
  Bus Selector4 : BusSelector  OutputSignals=Angular Rate ZED  OutputAsBus=on
  Bus Selector5 : BusSelector  OutputSignals=Quaternion ZED  OutputAsBus=on
  Gain1 : Gain  Gain=[-1,1,-1]
  Gain2 : Gain  Gain=[-1,1,-1]
  Gain3 : Gain  Gain=[1,-1,1,-1]
  MATLAB Function : MATLAB Function  TreatAsAtomicUnit=on
  MATLAB Function1 : MATLAB Function  TreatAsAtomicUnit=on
  Mux : Mux  Inputs=3
  Mux1 : Mux  Inputs=2
  Quaternion Conjugate : aerolibutil/Quaternion Conjugate
  Quaternion Conjugate1 : aerolibutil/Quaternion Conjugate
  Quaternion Inverse : aerolibutil/Quaternion Inverse
  Quaternion Inverse1 : aerolibutil/Quaternion Inverse
  IMU : Outport
  ZED : Outport  Port=2
  wires:
  Bus Selector/1 -> MATLAB Function/1(u)
  MATLAB Function/1(y) -> Quaternion Conjugate/1
  Quaternion Conjugate/1 -> Quaternion Inverse/1
  Quaternion Inverse/1 -> Acceleration to velocity/1(q), Mux/1  "qS2W"
  Bus Selector2/1 -> Acceleration to velocity/3(Angular Rate), Mux/3  "Angular Rate"
  Mux/1 -> IMU/1
  MATLAB Function1/1(y) -> Quaternion Conjugate1/1
  Quaternion Conjugate1/1 -> Quaternion Inverse1/1
  Acceleration to velocity ZED/1(vec_rot) -> ?
  Bus Selector5/1 -> Gain3/1
  y/1 -> Bus Selector4/1, Bus Selector3/1, Bus Selector5/1, Bus Selector2/1, Bus Selector1/1, Bus Selector/1
  Bus Selector3/1 -> Gain2/1  "Linear ACC ZED"
  Mux1/1 -> ZED/1
  SensorOn/1 -> Acceleration to velocity/4(SensorOn), Acceleration to velocity ZED/4(SensorOn)
  Quaternion Inverse1/1 -> Mux1/1, Acceleration to velocity ZED/1(q)  "qS2W"
  Bus Selector4/1 -> Gain1/1  "Angular Rate ZED"
  Bus Selector1/1 -> Acceleration to velocity/2(vec)
  Acceleration to velocity/1(vec_rot) -> Mux/2
  Gain3/1 -> MATLAB Function1/1(u)
  Gain2/1 -> Acceleration to velocity ZED/2(vec)
  Gain1/1 -> Mux1/2, Acceleration to velocity ZED/3(Angular Rate)

== system proc_control_lite/Subsystem ProcNav/DVL Measurements ==
  note: Mettre les vitesse dvl dans le frame Sous-marin
  DVL Velocity : Inport
  mecConst : Inport  Port=2
  Enable : EnablePort
  Bus Creator : BusCreator  Inputs=3
  Bus Selector : BusSelector  OutputSignals=dvl_rotation
  Bus Selector1 : BusSelector  OutputSignals=DVL Bot Velocity
  Bus Selector2 : BusSelector  OutputSignals=DVL Water Velocity
  Constant : Constant  Value=simulation.sensors.dvl.maxSpeedThres
  DVL2Ship : Subsystem
  MATLAB Function : MATLAB Function  TreatAsAtomicUnit=on
  Quaternion Rotation : aerolibutil/Quaternion Rotation
  Scope : Scope
  DVL Measurements : Outport
  wires:
  mecConst/1 -> Bus Selector/1
  DVL Velocity/1 -> Bus Selector1/1, Bus Selector2/1
  Bus Selector/1 -> DVL2Ship/1(dvl Rotation)  "<dvl_rotation>"
  Bus Selector1/1 -> MATLAB Function/1(vBot)  "<DVL Bot Velocity>"
  Bus Selector2/1 -> MATLAB Function/2(vWater)  "<DVL Water Velocity>"
  Constant/1 -> MATLAB Function/3(thres)
  MATLAB Function/1(v) -> Quaternion Rotation/2
  DVL2Ship/1(Quat) -> Quaternion Rotation/1
  Quaternion Rotation/1 -> Bus Creator/1, Scope/1  "Body Velocity"
  MATLAB Function/2(error) -> Bus Creator/2  "error"
  MATLAB Function/3(enable) -> Bus Creator/3  "enable"
  Bus Creator/1 -> DVL Measurements/1

== system proc_control_lite/Subsystem ProcNav/Depth Measurements ==
  note: Transformer la mesure du detph selon BF
  y : Inport
  mecConst : Inport  Port=2
  xhat : Inport  Port=3
  Enable : EnablePort
  Bus Selector : BusSelector  OutputSignals=Pressure Depth  OutputAsBus=on
  Bus Selector1 : BusSelector  OutputSignals=depth_pose
  Discrete Transfer Fcn : DiscreteTransferFcn  Numerator=[physics.thruster.a1 0 ]  Denominator="[1  physics.thruster.b0]"
  Discrete Derivative : simulink/Discrete/Discrete Derivative  gainval=1.0  ICPrevScaledInput=0.0  OutMin=[]  OutMax=[]  OutDataType=fixdt(1, 16)  OutScaling=2^-10  DoSatur=off
  Mux : Mux  Inputs=2
  Quaternion Rotation : aerolibutil/Quaternion Rotation
  Selector : Selector  InputPortWidth=10  IndexOptions=Index vector (dialog)  Indices=[1:4]  OutputSizes=1
  Selector1 : Selector  InputPortWidth=3  IndexOptions=Index vector (dialog)  Indices=[3]  OutputSizes=1
  Sum : Sum  Inputs=|+-
  Depth Measurements : Outport
  wires:
  y/1 -> Bus Selector/1
  Bus Selector/1 -> Sum/1  "pressure Depth"
  Sum/1 -> Mux/1, Discrete Derivative/1  "z position"
  xhat/1 -> Selector/1
  mecConst/1 -> Bus Selector1/1
  Selector/1 -> Quaternion Rotation/1
  Bus Selector1/1 -> Quaternion Rotation/2  "<depth_pose>"
  Quaternion Rotation/1 -> Selector1/1
  Selector1/1 -> Sum/2
  Mux/1 -> Depth Measurements/1
  Discrete Derivative/1 -> Discrete Transfer Fcn/1
  Discrete Transfer Fcn/1 -> Mux/2  "z velocity"

== system proc_control_lite/Subsystem ProcNav/Enabled Subsystem ==
  stateFuncArguments : Inport
  AHRS Mesurments : Inport  Port=2
  ZED : Inport  Port=3
  "DVL Measurements " : Inport  Port=4
  Depth Measurements : Inport  Port=5
  mecConst : Inport  Port=6
  Enable : EnablePort  StatesWhenEnabling=reset
  Extended Kalman Filter2 : sharedTrackingLibrary/Extended Kalman Filter  StateTransitionFcn=EkfNavStatesEq  HasStateTransitionJacobianFcn=off  HasAdditiveProcessNoise=Additive  ProcessNoise=kalman.Cx  HasTimeVaryingProcessNoise=off  HasStateTransitionFcnExtraArgument=1  InitialState=kalman.Xi  InitialStateCovariance=kalman.Ci  MeasurementFcn1=EkfNavAhrs  HasMeasurementJacobianFcn1=off  HasMeasurementEnablePort1=off  HasAdditiveMeasurementNoise1=Additive  MeasurementNoise1=kalman.Cimu  HasTimeVaryingMeasurementNoise1=off  HasMeasurementFcnExtraArgument1=0  HasMeasurementWrapping1=off  MeasurementFcn2=EkfNavDvl  HasMeasurementJacobianFcn2=off  HasMeasurementEnablePort2=on  HasAdditiveMeasurementNoise2=Additive  MeasurementNoise2=kalman.Cdvl  HasTimeVaryingMeasurementNoise2=off  HasMeasurementFcnExtraArgument2=0  HasMeasurementWrapping2=off  MeasurementFcn3=EkfNavDepth  HasMeasurementJacobianFcn3=off  HasMeasurementEnablePort3=off  HasAdditiveMeasurementNoise3=Additive  MeasurementNoise3=kalman.Cdepth  HasTimeVaryingMeasurementNoise3=off  HasMeasurementFcnExtraArgument3=0  HasMeasurementWrapping3=off  MeasurementFcn4=EkfNavZED  HasMeasurementJacobianFcn4=off  HasMeasurementEnablePort4=off  HasAdditiveMeasurementNoise4=Additive  MeasurementNoise4=kalman.CimuZED  HasTimeVaryingMeasurementNoise4=off  HasMeasurementFcnExtraArgument4=0  HasMeasurementWrapping4=off  MeasurementFcn5=myMeasurementFcn  HasMeasurementJacobianFcn5=off  HasMeasurementEnablePort5=off  HasAdditiveMeasurementNoise5=Additive  MeasurementNoise5=1  HasTimeVaryingMeasurementNoise5=off  HasMeasurementFcnExtraArgument5=0  HasMeasurementWrapping5=off  EnableMultirate=on  StateTransitionFcnSampleTime=simulink.procNav.sampletime  MeasurementFcn1SampleTime=simulink.procNav.imuDepth.sampletime  MeasurementFcn2SampleTime=simulink.procNav.dvl.sampletime  MeasurementFcn3SampleTime=simulation.sensors.depth.sampletime  MeasurementFcn4SampleTime=simulation.sensors.depth.sampletime  MeasurementFcn5SampleTime=1  UseCurrentEstimator=on  OutputStateCovariance=on  DataType=double  SampleTime=1  NumberOfMeasurements=3
  Scope : Scope
  Selector : Selector  InputPortWidth=2  IndexOptions=Index vector (dialog)  Indices=[1]  OutputSizes=1
  Subsystem : Subsystem
  Terminator : Terminator
  Zero-Order Hold1 : ZeroOrderHold  SampleTime=simulation.sensors.depth.sampletime
  xhat : Outport
  wires:
  stateFuncArguments/1 -> Extended Kalman Filter2/1
  AHRS Mesurments/1 -> Extended Kalman Filter2/2  "ahrs"
  Depth Measurements/1 -> Selector/1
  Selector/1 -> Zero-Order Hold1/1
  Zero-Order Hold1/1 -> Extended Kalman Filter2/5  "depth"
  Extended Kalman Filter2/1 -> xhat/1
  Extended Kalman Filter2/2 -> Scope/1
  ZED/1 -> Terminator/1
  "DVL Measurements "/1 -> Subsystem/2(In2)
  mecConst/1 -> Subsystem/1(mecConst)
  Subsystem/1(Out1) -> Extended Kalman Filter2/3
  Subsystem/2(y1) -> Extended Kalman Filter2/4

== system proc_control_lite/Subsystem ProcNav/Reset Logic ==
  In1 : Inport
  2 : Inport  Port=2
  AND : Logic  IconShape=distinctive  AllPortsSameDT=off  OutDataTypeStr=boolean
  NOT : Logic  Operator=NOT  IconShape=distinctive  AllPortsSameDT=off  OutDataTypeStr=boolean
  Out1 : Outport
  wires:
  2/1 -> AND/2
  In1/1 -> NOT/1
  NOT/1 -> AND/1
  AND/1 -> Out1/1

== system proc_control_lite/Subsystem ProcNav/State function arguments ==
  thrust : Inport
  mecConst : Inport  Port=2
  Bus Selector : BusSelector  OutputSignals=mass,volume,sub_height,I,rg,rb,cdl,cdq,added_mass,rho,g  OutputAsBus=on
  Bus Selector1 : BusSelector  OutputSignals=thrusters  OutputAsBus=on
  Bus to Vector : BusToVector
  Constant : Constant  Value=[0,0,0,0,0,0,0,0]
  Delay : Delay  DelayLength=1  InitialCondition=[0,0,0,0,0,0,0,0]
  Display : Display
  Mux : Mux
  Probe : Probe  ProbeSignalDimensions=on
  Reshape : Reshape
  Transpose : Math  Operator=transpose
  Zero-Order Hold : ZeroOrderHold  SampleTime=simulink.procNav.sampletime
  stateFuncArguments : Outport
  wires:
  mecConst/1 -> Bus Selector/1, Bus Selector1/1
  Bus Selector1/1 -> Transpose/1
  Constant/1 -> Probe/1, Delay/1
  Delay/1 -> Zero-Order Hold/1
  Bus Selector/1 -> Bus to Vector/1
  Bus to Vector/1 -> Mux/3
  Transpose/1 -> Reshape/1
  Probe/1 -> Mux/1
  Zero-Order Hold/1 -> Mux/2
  Reshape/1 -> Mux/4, Display/1
  Mux/1 -> stateFuncArguments/1

== system proc_control_lite/Subsystem ProcNav/mux2Bus ==
  xhat : Inport
  Bus Creator : BusCreator  Inputs=5
  Quaternion Inverse : aerolibutil/Quaternion Inverse
  Scope{,1..3} (4 alike) : Scope
  Selector : Selector  InputPortWidth=13  IndexOptions=Index vector (dialog)  Indices=[1:3]  OutputSizes=1
  Selector1 : Selector  InputPortWidth=13  IndexOptions=Index vector (dialog)  Indices=[4:7]  OutputSizes=1
  Selector2 : Selector  InputPortWidth=13  IndexOptions=Index vector (dialog)  Indices=[8:10]  OutputSizes=1
  Selector3 : Selector  InputPortWidth=13  IndexOptions=Index vector (dialog)  Indices=[11:13]  OutputSizes=1
  states : Outport
  wires:
  xhat/1 -> Selector3/1, Selector2/1, Selector1/1, Selector/1
  Selector/1 -> Scope/1, Bus Creator/1  "WorldPosition"
  Selector3/1 -> Scope3/1, Bus Creator/5  "Angular Rate"
  Selector1/1 -> Scope1/1, Quaternion Inverse/1, Bus Creator/2  "qS2W"
  Selector2/1 -> Scope2/1, Bus Creator/4  "Body Velocity"
  Bus Creator/1 -> states/1
  Quaternion Inverse/1 -> Bus Creator/3  "qW2S"

== system proc_control_lite/Subsystem Trajectory/IDLE ==
  Action Port : ActionPort  ActionPortLabel=default:
  Bus Creator : BusCreator  Inputs=4
  Constant : Constant  Value=[0,0,0.3,1,0,0,0,0,0,0,0,0,0]
  Constant1 : Constant  Value=MPC.p
  Constant2 : Constant  Value=false
  Constant3 : Constant  Value=false
  MATLAB Function : MATLAB Function  TreatAsAtomicUnit=on
  Selector : Selector  InputPortWidth=13  IndexOptions=Index vector (dialog)  Indices=[1:7]  OutputSizes=1
  Transpose : Math  Operator=transpose
  y : Outport
  wires:
  Constant/1 -> Transpose/1
  Transpose/1 -> Selector/1, MATLAB Function/1(matrix)
  Constant1/1 -> MATLAB Function/2(p)
  MATLAB Function/1(y) -> Bus Creator/1  "Reference"
  Selector/1 -> Bus Creator/4  "target"
  Constant2/1 -> Bus Creator/2  "isReached"
  Constant3/1 -> Bus Creator/3  "isTrajDone"
  Bus Creator/1 -> y/1

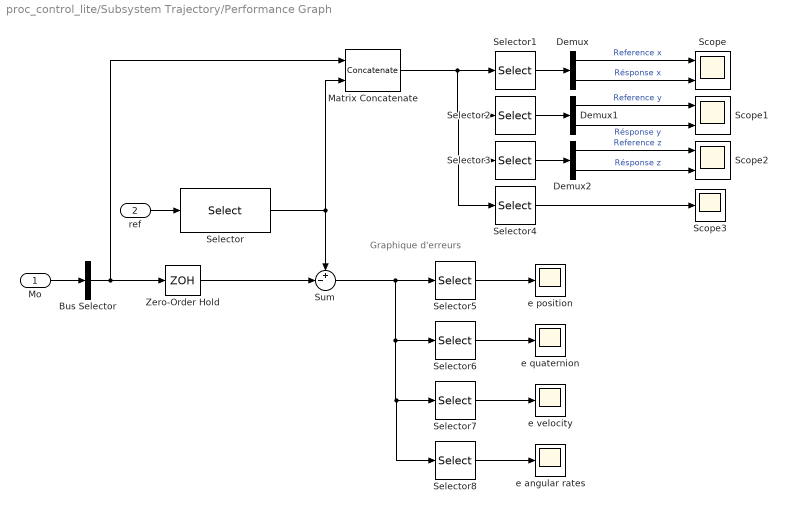
== system proc_control_lite/Subsystem Trajectory/Performance Graph ==
  note: Graphique d'erreurs
  Mo : Inport
  ref : Inport  Port=2
  Bus Selector : BusSelector  OutputSignals=WorldPosition,qS2W,Body Velocity,Angular Rate  OutputAsBus=on
  Demux : Demux  Outputs=2
  Demux1 : Demux  Outputs=2
  Demux2 : Demux  Outputs=2
  Matrix Concatenate : Concatenate  Mode=Multidimensional array
  Scope : Scope  NumInputPorts=2
  Scope1 : Scope  NumInputPorts=2
  Scope2 : Scope  NumInputPorts=2
  Scope3 : Scope
  Selector : Selector  NumberOfDimensions=2  InputPortWidth=3  IndexOptions=Index vector (dialog),Index vector (dialog)  Indices=[1],[1:13]  OutputSizes=1,1
  Selector1 : Selector  NumberOfDimensions=2  InputPortWidth=3  IndexOptions=Index vector (dialog),Index vector (dialog)  Indices=[1:2],1  OutputSizes=1,1
  Selector2 : Selector  NumberOfDimensions=2  InputPortWidth=3  IndexOptions=Index vector (dialog),Index vector (dialog)  Indices=[1:2],2  OutputSizes=1,1
  Selector3 : Selector  NumberOfDimensions=2  InputPortWidth=3  IndexOptions=Index vector (dialog),Index vector (dialog)  Indices=[1:2],3  OutputSizes=1,1
  Selector4 : Selector  NumberOfDimensions=2  InputPortWidth=3  IndexOptions=Index vector (dialog),Index vector (dialog)  Indices=[1:2],[4:7]  OutputSizes=1,1
  Selector5 : Selector  InputPortWidth=13  IndexOptions=Index vector (dialog)  Indices=[1:3]  OutputSizes=1
  Selector6 : Selector  InputPortWidth=13  IndexOptions=Index vector (dialog)  Indices=[4:7]  OutputSizes=1
  Selector7 : Selector  InputPortWidth=13  IndexOptions=Index vector (dialog)  Indices=[8:10]  OutputSizes=1
  Selector8 : Selector  InputPortWidth=13  IndexOptions=Index vector (dialog)  Indices=[10:13]  OutputSizes=1
  Sum : Sum  Inputs=+-|
  Zero-Order Hold : ZeroOrderHold  SampleTime=-1
  e angular rates : Scope
  e position : Scope
  e quaternion : Scope
  e velocity : Scope
  wires:
  Mo/1 -> Bus Selector/1
  Bus Selector/1 -> Matrix Concatenate/1, Zero-Order Hold/1
  Zero-Order Hold/1 -> Sum/2
  ref/1 -> Selector/1
  Selector/1 -> Sum/1, Matrix Concatenate/2
  Matrix Concatenate/1 -> Selector4/1, Selector3/1, Selector2/1, Selector1/1
  Selector1/1 -> Demux/1
  Selector2/1 -> Demux1/1
  Selector3/1 -> Demux2/1
  Demux/1 -> Scope/1  "Reference x"
  Demux/2 -> Scope/2  "Résponse x"
  Demux1/1 -> Scope1/1  "Reference y"
  Demux1/2 -> Scope1/2  "Résponse y"
  Demux2/1 -> Scope2/1  "Reference z"
  Demux2/2 -> Scope2/2  "Résponse z"
  Selector4/1 -> Scope3/1
  Sum/1 -> Selector8/1, Selector7/1, Selector6/1, Selector5/1
  Selector5/1 -> e position/1
  Selector6/1 -> e quaternion/1
  Selector7/1 -> e velocity/1
  Selector8/1 -> e angular rates/1
